simulink model "model_3"  (R2022a)
settings: Solver=VariableStepAuto  StartTime=0.0  StopTime=30  RelTol=1e-3
values from neighbouring files (symbols this model uses):
  A = [6, 7, -4, 8; 0, 9, 0, 15; 10, 13, -6, 19; 0, -6, 0, -9]    [task_2.m]
  C = eye(4)    [task_2.m]
  x0 = [1; -1; 1; -1]    [task_2.m]
undefined symbols (not defined in the file or in its folder): L_1, L_2, L_3, x_0
settings Model: Creator=vital  LastModifiedBy=Family
settings DebuggingCC: UnconnectedInputMsg=warning  UnconnectedOutputMsg=warning  UnconnectedLineMsg=warning
settings RTWCC: DLArmComputeVersion=19.05

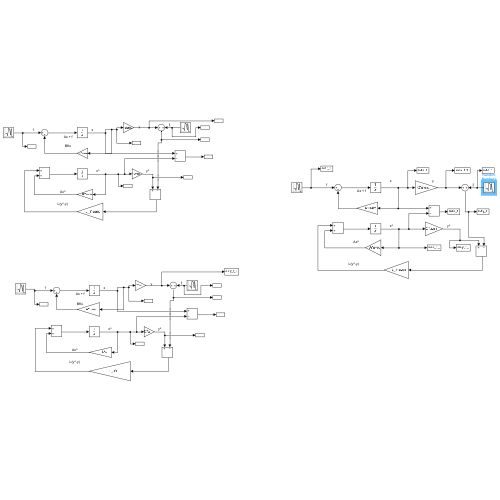
[thumbnail: Simulink's stored preview of the top-level diagram]
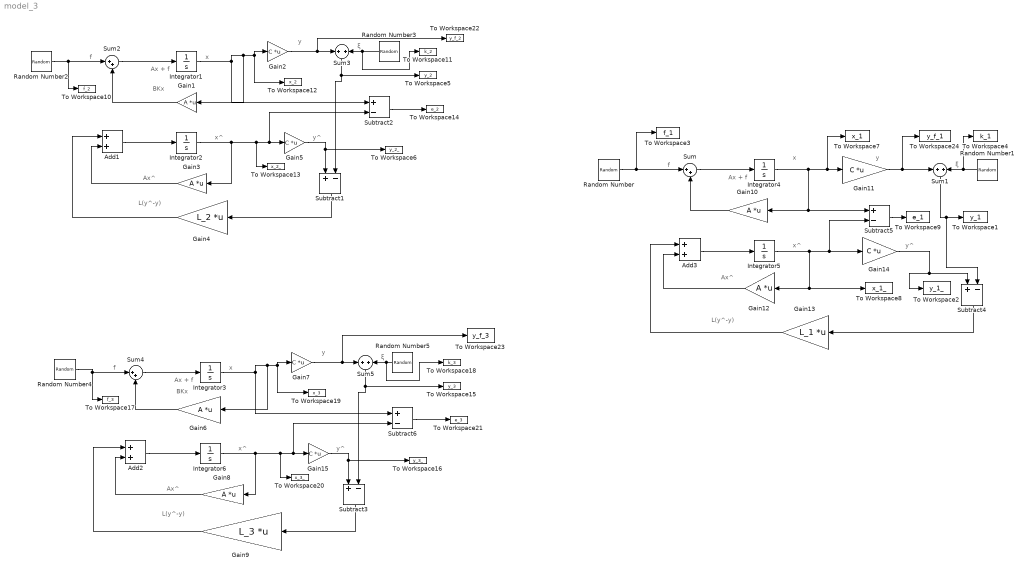
== system model_3 ==
  note: ξ
  note: f
  note: y
  note: Ax^
  note: Ax + f
  note: x
  note: y^
  note: x^
  note: L(y^-y)
  note: y
  note: y^
  note: Ax + f
  note: f
  note: ξ
  note: x
  note: L(y^-y)
  note: x^
  note: BKx
  note: Ax^
  note: y
  note: y^
  note: Ax + f
  note: f
  note: ξ
  note: x
  note: L(y^-y)
  note: x^
  note: BKx
  note: Ax^
  Add1 : Sum
  Add2 : Sum
  Add3 : Sum
  Gain{1,3,6,10,12} (5 alike) : Gain  Gain=A  Multiplication=Matrix(K*u) (u vector)
  Gain{2,5,11,14} (4 alike) : Gain  Gain=C  Multiplication=Matrix(K*u) (u vector)
  Gain13 : Gain  Gain=L_1  Multiplication=Matrix(K*u) (u vector)
  Gain15 : Gain  Gain=C  Multiplication=Matrix(K*u)
  Gain4 : Gain  Gain=L_2  Multiplication=Matrix(K*u) (u vector)
  Gain7 : Gain  Gain=C  Multiplication=Matrix(K*u)
  Gain8 : Gain  Gain=A  Multiplication=Matrix(K*u)
  Gain9 : Gain  Gain=L_3  Multiplication=Matrix(K*u)
  Integrator1 : Integrator  InitialCondition=x0
  Integrator2 : Integrator  InitialCondition=x_0
  Integrator3 : Integrator  InitialCondition=x0
  Integrator4 : Integrator  InitialCondition=x0
  Integrator5 : Integrator  InitialCondition=x_0
  Integrator6 : Integrator  InitialCondition=x_0
  Random Number : RandomNumber  Variance=50  Seed=[1; 2; 3; 4]  SampleTime=0000.1
  Random Number1 : RandomNumber  Variance=50  Seed=[5 ; 6]  SampleTime=00000.1
  Random Number2 : RandomNumber  Variance=50  Seed=[7; 8; 9; 10]  SampleTime=0000.1
  Random Number3 : RandomNumber  Variance=50  Seed=[11 ; 12]  SampleTime=0000.1
  Random Number4 : RandomNumber  Variance=50  Seed=[13; 14; 15; 16]  SampleTime=0000.1
  Random Number5 : RandomNumber  Variance=50  Seed=[17; 18]  SampleTime=0000.1
  Subtract{1..6} (6 alike) : Sum  Inputs=+-
  Sum : Sum  Inputs=|++
  Sum1 : Sum  Inputs=+|+
  Sum2 : Sum  Inputs=|++
  Sum3 : Sum  Inputs=+|+
  Sum4 : Sum  Inputs=|++
  Sum5 : Sum  Inputs=+|+
  To Workspace1 : ToWorkspace  VariableName=y_1  SaveFormat=Timeseries  SampleTime=-1
  To Workspace10 : ToWorkspace  VariableName=f_2  SaveFormat=Timeseries  SampleTime=-1
  To Workspace11 : ToWorkspace  VariableName=k_2  SaveFormat=Timeseries  SampleTime=-1
  To Workspace12 : ToWorkspace  VariableName=x_2  SaveFormat=Timeseries  SampleTime=0.0001
  To Workspace13 : ToWorkspace  VariableName=x_2_  SaveFormat=Timeseries  SampleTime=-1
  To Workspace14 : ToWorkspace  VariableName=e_2  SaveFormat=Timeseries  SampleTime=-1
  To Workspace15 : ToWorkspace  VariableName=y_3  SaveFormat=Timeseries  SampleTime=-1
  To Workspace16 : ToWorkspace  VariableName=y_3_  SaveFormat=Timeseries  SampleTime=-1
  To Workspace17 : ToWorkspace  VariableName=f_3  SaveFormat=Timeseries  SampleTime=-1
  To Workspace18 : ToWorkspace  VariableName=k_3  SaveFormat=Timeseries  SampleTime=-1
  To Workspace19 : ToWorkspace  VariableName=x_3  SaveFormat=Timeseries  SampleTime=0.0001
  To Workspace2 : ToWorkspace  VariableName=y_1_  SaveFormat=Timeseries  SampleTime=-1
  To Workspace20 : ToWorkspace  VariableName=x_3_  SaveFormat=Timeseries  SampleTime=-1
  To Workspace21 : ToWorkspace  VariableName=e_3  SaveFormat=Timeseries  SampleTime=-1
  To Workspace22 : ToWorkspace  VariableName=y_f_2  SaveFormat=Timeseries  SampleTime=-1
  To Workspace23 : ToWorkspace  VariableName=y_f_3  SaveFormat=Timeseries  SampleTime=-1
  To Workspace24 : ToWorkspace  VariableName=y_f_1  SaveFormat=Timeseries  SampleTime=-1
  To Workspace3 : ToWorkspace  VariableName=f_1  SaveFormat=Timeseries  SampleTime=-1
  To Workspace4 : ToWorkspace  VariableName=k_1  SaveFormat=Timeseries  SampleTime=-1
  To Workspace5 : ToWorkspace  VariableName=y_2  SaveFormat=Timeseries  SampleTime=-1
  To Workspace6 : ToWorkspace  VariableName=y_2_  SaveFormat=Timeseries  SampleTime=-1
  To Workspace7 : ToWorkspace  VariableName=x_1  SaveFormat=Timeseries  SampleTime=0.00001
  To Workspace8 : ToWorkspace  VariableName=x_1_  SaveFormat=Timeseries  SampleTime=-1
  To Workspace9 : ToWorkspace  VariableName=e_1  SaveFormat=Timeseries  SampleTime=-1
  wires:
  Gain10/1 -> Sum/2
  Integrator4/1 -> Gain10/1, Subtract5/1, To Workspace7/1, Gain11/1
  Integrator5/1 -> To Workspace8/1, Gain12/1, Subtract5/2, Gain14/1
  Add3/1 -> Integrator5/1
  Gain14/1 -> Subtract4/1, To Workspace2/1
  Gain12/1 -> Add3/2
  Subtract4/1 -> Gain13/1
  Gain13/1 -> Add3/1
  Subtract5/1 -> To Workspace9/1
  Random Number/1 -> Sum/1, To Workspace3/1
  Sum/1 -> Integrator4/1
  Sum1/1 -> Subtract4/2, To Workspace1/1
  Random Number1/1 -> Sum1/2, To Workspace4/1
  Random Number3/1 -> To Workspace11/1, Sum3/2
  Gain4/1 -> Add1/1
  Gain2/1 -> To Workspace22/1, Sum3/1
  Gain5/1 -> To Workspace6/1, Subtract1/1
  Sum3/1 -> Subtract1/2, To Workspace5/1
  Add1/1 -> Integrator2/1
  Subtract2/1 -> To Workspace14/1
  Sum2/1 -> Integrator1/1
  Integrator1/1 -> To Workspace12/1, Gain2/1, Gain1/1, Subtract2/1
  Subtract1/1 -> Gain4/1
  Gain3/1 -> Add1/2
  Random Number2/1 -> To Workspace10/1, Sum2/1
  Gain1/1 -> Sum2/2
  Integrator2/1 -> Gain3/1, To Workspace13/1, Subtract2/2, Gain5/1
  Random Number5/1 -> To Workspace18/1, Sum5/2
  Gain9/1 -> Add2/1
  Gain7/1 -> To Workspace23/1, Sum5/1
  Gain15/1 -> To Workspace16/1, Subtract3/1
  Sum5/1 -> Subtract3/2, To Workspace15/1
  Add2/1 -> Integrator6/1
  Subtract6/1 -> To Workspace21/1
  Sum4/1 -> Integrator3/1
  Integrator3/1 -> To Workspace19/1, Gain7/1, Gain6/1, Subtract6/1
  Subtract3/1 -> Gain9/1
  Gain8/1 -> Add2/2
  Random Number4/1 -> To Workspace17/1, Sum4/1
  Gain6/1 -> Sum4/2
  Integrator6/1 -> Gain8/1, To Workspace20/1, Subtract6/2, Gain15/1
  Gain11/1 -> To Workspace24/1, Sum1/1
